simulink model "zz_sim_PIDController_eg2"  (R2021b)
settings: Solver=VariableStepAuto  StartTime=0.0  StopTime=10.0  RelTol=1e-3
settings Model: Creator=Samir  LastModifiedBy=Samir
settings SolverCC: ZeroCrossAlgorithm=Adaptive
settings DebuggingCC: IgnoredZcDiagnostic=none

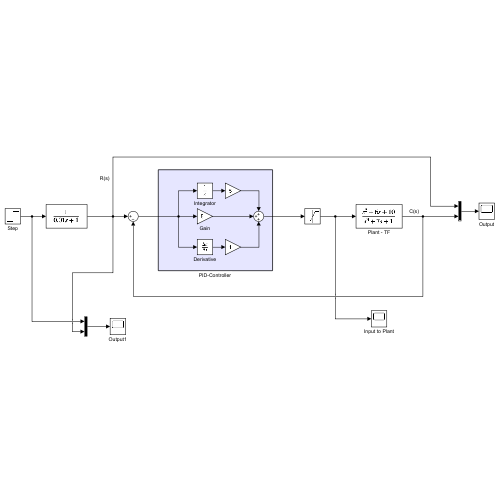
[thumbnail: Simulink's stored preview of the top-level diagram]
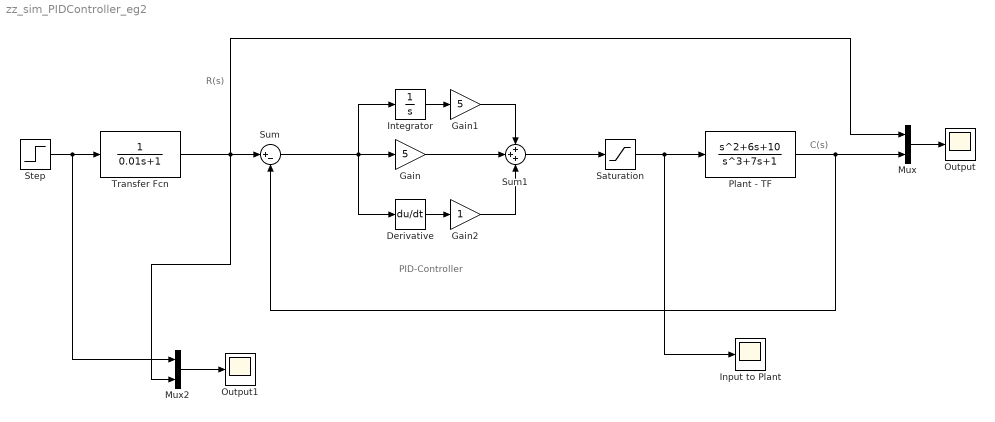
== system zz_sim_PIDController_eg2 ==
  note: C(s)
  note: R(s)
  note: PID-Controller
  Derivative : Derivative
  Gain : Gain  Gain=5
  Gain1 : Gain  Gain=5
  Gain2 : Gain
  Input to Plant : Scope
  Integrator : Integrator
  Mux : Mux  Inputs=2
  Mux2 : Mux  Inputs=2
  Output : Scope
  Output1 : Scope
  Plant - TF : TransferFcn  Numerator=[1 6 10]  Denominator=[1 0 7 1]
  Saturation : Saturate  UpperLimit=7  LowerLimit=-7
  Step : Step  SampleTime=0
  Sum : Sum  Inputs=|+-
  Sum1 : Sum  Inputs=+++
  Transfer Fcn : TransferFcn  Denominator=[0.01 1]
  wires:
  Plant - TF/1 -> Mux/2, Sum/2
  Step/1 -> Mux2/1, Transfer Fcn/1
  Sum/1 -> Derivative/1, Integrator/1, Gain/1
  Mux/1 -> Output/1
  Integrator/1 -> Gain1/1
  Gain/1 -> Sum1/2
  Sum1/1 -> Saturation/1
  Gain1/1 -> Sum1/1
  Derivative/1 -> Gain2/1
  Gain2/1 -> Sum1/3
  Transfer Fcn/1 -> Mux2/2, Mux/1, Sum/1
  Saturation/1 -> Input to Plant/1, Plant - TF/1
  Mux2/1 -> Output1/1
